simulink model "Zad1"  (R2018a)
settings: Solver=ode4  StartTime=0.0  StopTime=10.0  FixedStep=2^-7  RelTol=1e-3
libraries: simulink x2
settings Model: Creator=Koala  LastModifiedBy=Koala

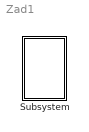
== system Zad1 ==
  Subsystem : Subsystem  mask{vx=15, x0=0, vy=0, y0=5, M=100, G=9.81, R=2, Rs=0.2}

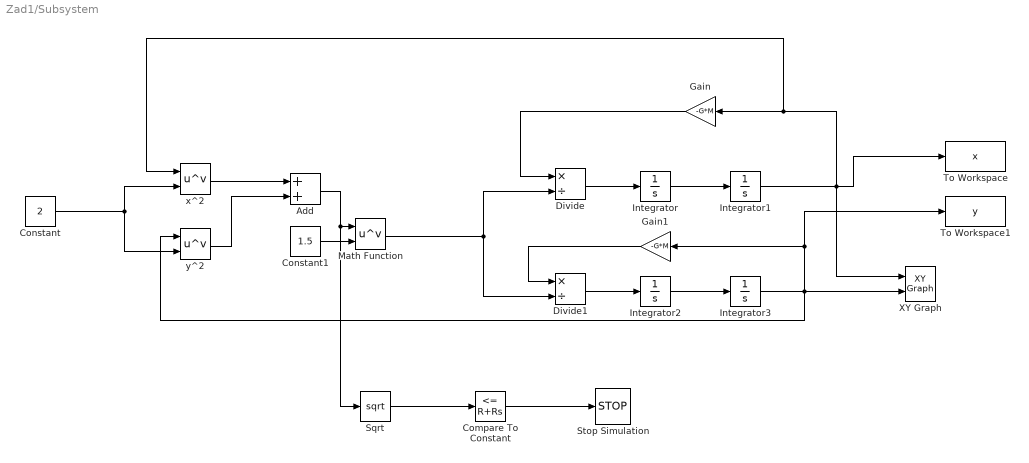
== system Zad1/Subsystem ==
  Add : Sum
  Compare To Constant : simulink/Logic and Bit Operations/Compare To Constant  relop=<=  const=R+Rs  OutDataTypeStr=boolean
  Constant : Constant  Value=2
  Constant1 : Constant  Value=1.5
  Divide : Product  Inputs=*/
  Divide1 : Product  Inputs=*/
  Gain : Gain  Gain=-G*M
  Gain1 : Gain  Gain=-G*M
  Integrator : Integrator  InitialCondition=vx
  Integrator1 : Integrator  InitialCondition=x0
  Integrator2 : Integrator  InitialCondition=vy
  Integrator3 : Integrator  InitialCondition=y0
  Math Function : Math  Operator=pow  SaturateOnIntegerOverflow=on
  Sqrt : Sqrt  SaturateOnIntegerOverflow=on
  Stop Simulation : Stop
  To Workspace : ToWorkspace  VariableName=x  SampleTime=-1
  To Workspace1 : ToWorkspace  VariableName=y  SampleTime=-1
  XY Graph : simulink/Sinks/XY Graph  xmin=-10  xmax=10  ymin=-10  ymax=10  st=-1
  x^2 : Math  Operator=pow  SaturateOnIntegerOverflow=on
  y^2 : Math  Operator=pow  SaturateOnIntegerOverflow=on
  wires:
  Integrator1/1 -> To Workspace/1, x^2/1, Gain/1, XY Graph/1
  Gain/1 -> Divide/1
  Divide/1 -> Integrator/1
  Math Function/1 -> Divide/2, Divide1/2
  Integrator2/1 -> Integrator3/1
  Integrator3/1 -> To Workspace1/1, Gain1/1, XY Graph/2, y^2/1
  Divide1/1 -> Integrator2/1
  Constant1/1 -> Math Function/2
  x^2/1 -> Add/1
  Constant/1 -> x^2/2, y^2/2
  Integrator/1 -> Integrator1/1
  y^2/1 -> Add/2
  Add/1 -> Sqrt/1, Math Function/1
  Gain1/1 -> Divide1/1
  Sqrt/1 -> Compare To Constant/1
  Compare To Constant/1 -> Stop Simulation/1
